simulink model "DC_MOTOR"  (R2020b)
settings: Solver=ode15s  StartTime=0.0  StopTime=0.2  RelTol=1e-3
values from neighbouring files (symbols this model uses):
  b = 3.5077E-6    (= 3.5077e-06)    [variable.m]
  J = 3.228E-6    (= 3.228e-06)    [variable.m]
  K = 0.0274    [variable.m]
  L = 2.74e-4    (= 0.000274)    [variable.m]
  R = 4    [variable.m]
settings Model: Creator=nadee  LastModifiedBy=sonal
settings DataIOCC: SaveOutput=off  SaveTime=off

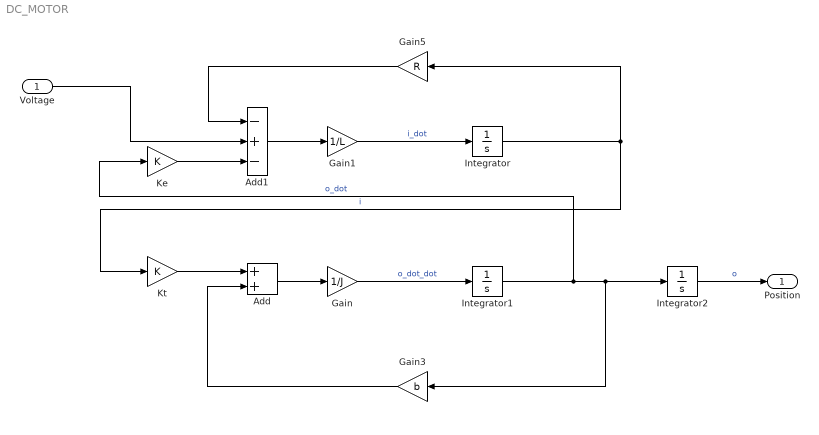
== system DC_MOTOR ==
  Voltage : Inport  OutDataTypeStr=double  PortDimensions=1  SampleTime=0
  Add : Sum
  Add1 : Sum  Inputs=-+-
  Gain : Gain  Gain=1/J
  Gain1 : Gain  Gain=1/L
  Gain3 : Gain  Gain=b
  Gain5 : Gain  Gain=R
  Integrator : Integrator
  Integrator1 : Integrator
  Integrator2 : Integrator
  Ke : Gain  Gain=K
  Kt : Gain  Gain=K
  Position : Outport  OutDataTypeStr=double  PortDimensions=1  SampleTime=0
  wires:
  Add/1 -> Gain/1
  Gain3/1 -> Add/2
  Integrator1/1 -> Ke/1, Gain3/1, Integrator2/1  "o_dot"
  Add1/1 -> Gain1/1
  Kt/1 -> Add/1
  Gain5/1 -> Add1/1
  Integrator/1 -> Kt/1, Gain5/1  "i"
  Gain/1 -> Integrator1/1  "o_dot_dot"
  Gain1/1 -> Integrator/1  "i_dot"
  Ke/1 -> Add1/3
  Voltage/1 -> Add1/2
  Integrator2/1 -> Position/1  "o"
